simulink model "modelo_electromagnetico_completo"  (R2023b)
settings: Solver=VariableStepAuto  StartTime=0.0  StopTime=10.0  RelTol=1e-3
values from neighbouring files (symbols this model uses):
  L_d = 6.6 * 10^(-3)    (= 0.0066)    [polos_y_ceros.m]    (also in var1.m)
  L_ls = 0.8 * 10^(-3)    (= 0.0008)    [polos_y_ceros.m]    (also in var1.m)
  L_q = 5.8 * 10^(-3)    (= 0.0058)    [polos_y_ceros.m]    (also in var1.m)
  lambda_m = 0.016    [polos_y_ceros.m]    (also in var1.m)
  P_p = 3    [polos_y_ceros.m]    (also in var1.m)
settings Model: Creator=tomas  LastModifiedBy=tomas

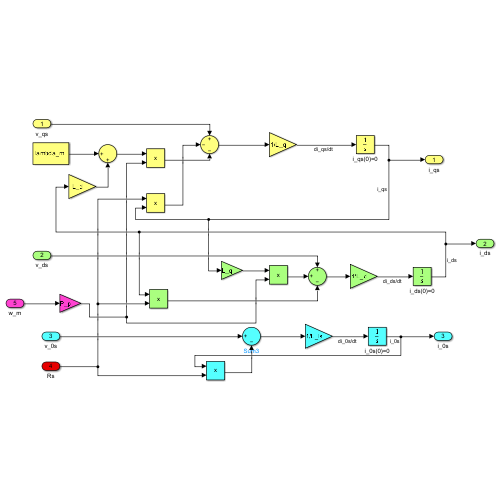
[thumbnail: Simulink's stored preview of the top-level diagram]
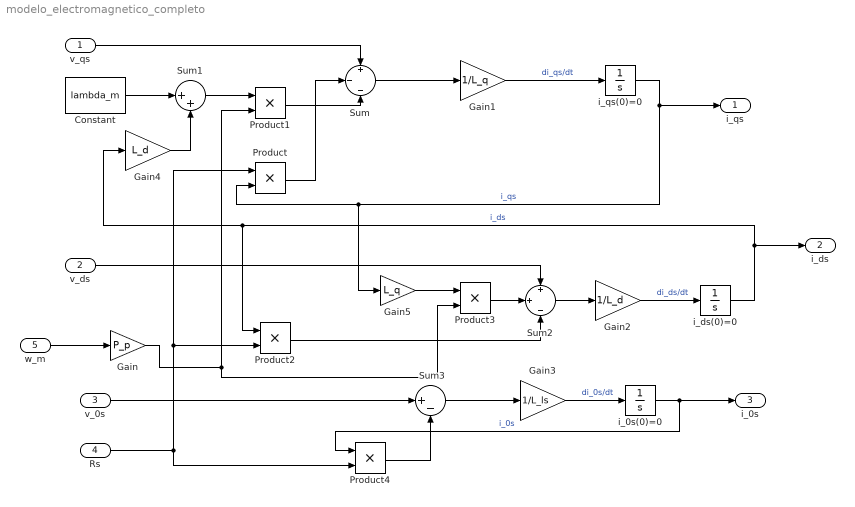
== system modelo_electromagnetico_completo ==
  v_qs : Inport
  v_ds : Inport  Port=2
  v_0s : Inport  Port=3
  Rs : Inport  Port=4
  w_m : Inport  Port=5
  Constant : Constant  Value=lambda_m
  Gain : Gain  Gain=P_p
  Gain1 : Gain  Gain=1/L_q
  Gain2 : Gain  Gain=1/L_d
  Gain3 : Gain  Gain=1/L_ls
  Gain4 : Gain  Gain=L_d
  Gain5 : Gain  Gain=L_q
  Product{,1..4} (5 alike) : Product
  Sum : Sum  Inputs=+|-|-
  Sum1 : Sum  Inputs=|++
  Sum2 : Sum  Inputs=+|+|-
  Sum3 : Sum  Inputs=|+-
  i_0s(0)=0 : Integrator
  i_ds(0)=0 : Integrator
  i_qs(0)=0 : Integrator
  i_qs : Outport
  i_ds : Outport  Port=2
  i_0s : Outport  Port=3
  wires:
  Gain1/1 -> i_qs(0)=0/1  "di_qs/dt"
  v_qs/1 -> Sum/1
  Product/1 -> Sum/2
  Rs/1 -> Product2/2, Product/1, Product4/2
  i_qs(0)=0/1 -> Gain5/1, Product/2, i_qs/1  "i_qs"
  Constant/1 -> Sum1/1
  Gain2/1 -> i_ds(0)=0/1  "di_ds/dt"
  Sum1/1 -> Product1/1
  w_m/1 -> Gain/1
  Gain/1 -> Product3/2, Product1/2
  Product1/1 -> Sum/3
  Sum/1 -> Gain1/1
  i_ds(0)=0/1 -> Product2/1, Gain4/1, i_ds/1  "i_ds"
  Gain4/1 -> Sum1/2
  Product2/1 -> Sum2/3
  Gain5/1 -> Product3/1
  Sum2/1 -> Gain2/1
  v_ds/1 -> Sum2/1
  Product3/1 -> Sum2/2
  Gain3/1 -> i_0s(0)=0/1  "di_0s/dt"
  v_0s/1 -> Sum3/1
  Product4/1 -> Sum3/2
  i_0s(0)=0/1 -> Product4/1, i_0s/1  "i_0s"
  Sum3/1 -> Gain3/1
